simulink model "sim_tvt_2025_pos_ctrl"  (R2020a)
settings: Solver=ode4  StartTime=0.0  StopTime=30.0  FixedStep=0.01  RelTol=1e-3
values from neighbouring files (symbols this model uses):
  alfa = 0.02    [init_tvt_2025_pos_ctrl.m]
  alfa_theta = 20    [init_tvt_2025_pos_ctrl.m]
  alfa_theta_obs = 100    [init_tvt_2025_pos_ctrl.m]
  c0 = 0.1    [init_tvt_2025_pos_ctrl.m]
  c1_diff_sigma_bar_v = diag([25; 30; 20])    [init_tvt_2025_pos_ctrl.m]
  c1v = diag([5.8; 6.5; 6.5])    [init_tvt_2025_pos_ctrl.m]
  c2_diff_sigma_bar_v = diag([50; 50; 10])    [init_tvt_2025_pos_ctrl.m]
  c2v = diag([5.8; 6.5; 6.5])    [init_tvt_2025_pos_ctrl.m]
  c3_diff_sigma_bar_v = diag([15; 15; 10])    [init_tvt_2025_pos_ctrl.m]
  c3v = diag([4.8; 6.4; 6.0])    [init_tvt_2025_pos_ctrl.m]
  delta_p_i_0 = zeros(3, NF)    [init_tvt_2025_pos_ctrl.m]
  delta_v_i_0 = zeros(3, NF)    [init_tvt_2025_pos_ctrl.m]
  dp_aa_t = 0.2 * ones(3, 5) + ( 1.0 - 0.2 ) * rand(3, 5)    [init_tvt_2025_pos_ctrl.m]
  dp_ff_t = [ 0.4 * ones(1, 5) + ( 1.0 - 0.4 ) * rand(1, 5);                      0.4 * ones(1, 5) + ( 1.0 - 0.4 ) * rand(1, 5);                      0.2 * ones(1, 5) + ( 0.6 - 0.2 ) * rand(1, 5) ]    [init_tvt_2025_pos_ctrl.m]
  dp_phi_t = ( - pi / 2 ) * ones(3, 5) + ( pi / 2 - ( - pi / 2 ) ) * rand(3, 5)    [init_tvt_2025_pos_ctrl.m]
  eps0 = [0.05; 0.01; 0.01]    [init_tvt_2025_pos_ctrl.m]
  eta_ld_hat_init = zeros(3,NF)    [init_tvt_2025_pos_ctrl.m]
  etai_0 = zeros(3,5)    [init_tvt_2025_pos_ctrl.m]
  gamma0 = diag([1, 1, 1])    [init_tvt_2025_pos_ctrl.m]
  k_phi = diag([10, 10, 10])    [init_tvt_2025_pos_ctrl.m]
  k_theta = diag([5, 5, 5])    [init_tvt_2025_pos_ctrl.m]
  kai0 = [15; 10; 10]    [init_tvt_2025_pos_ctrl.m]
  kai_1_t = 0.02    [init_tvt_2025_pos_ctrl.m]
  kai_3_t = 0.1    [init_tvt_2025_pos_ctrl.m]
  ksi_ld_hat_init = zeros(3,NF)    [init_tvt_2025_pos_ctrl.m]
  ksii_0 = zeros(3,5)    [init_tvt_2025_pos_ctrl.m]
  l1v = diag([20; 20; 20])    [init_tvt_2025_pos_ctrl.m]
  l2v = diag([30; 30; 30])    [init_tvt_2025_pos_ctrl.m]
  lam0 = [15; 10; 10]    [init_tvt_2025_pos_ctrl.m]
  lam1 = diag([5,5,5])    [init_tvt_2025_pos_ctrl.m]
  lam2 = diag([5,5,5])    [init_tvt_2025_pos_ctrl.m]
  lam3 = diag([5,5,5])    [init_tvt_2025_pos_ctrl.m]
  lam4 = diag([5,5,5])    [init_tvt_2025_pos_ctrl.m]
  Lamd_diff_sigma_bar_v = 0.5    [init_tvt_2025_pos_ctrl.m]
  mass_i = zeros(1,NF)    [init_tvt_2025_pos_ctrl.m]
  Mii = diag([1;0;0;0;1])    [init_tvt_2025_pos_ctrl.m]
  pos0 = zeros(3, 1)    [init_tvt_2025_pos_ctrl.m]
  pos_bar_init = zeros(3,NF)    [init_tvt_2025_pos_ctrl.m]
  PZ0 = P0(3)    [init_tvt_2025_pos_ctrl.m]
  PZ1 = 10    [init_tvt_2025_pos_ctrl.m]
  Qci_init = repmat([1;0;0;0],1,NF)    [init_tvt_2025_pos_ctrl.m]
  R0 = 4    [init_tvt_2025_pos_ctrl.m]
  R1 = 8    [init_tvt_2025_pos_ctrl.m]
  Rx2 = 10    [init_tvt_2025_pos_ctrl.m]
  Ry2 = 6    [init_tvt_2025_pos_ctrl.m]
  Rz2 = 4    [init_tvt_2025_pos_ctrl.m]
  T0 = 0    [init_tvt_2025_pos_ctrl.m]
  T1 = tseq1    (= 10)    [init_tvt_2025_pos_ctrl.m]
  T12 = tseq1 + tseq12    (= 20)    [init_tvt_2025_pos_ctrl.m]
  T2 = tseq1 + tseq12 + tseq2    (= 30)    [init_tvt_2025_pos_ctrl.m]
  theta0 = ( 2 / 5 ) * pi    (= 1.25663706144)    [init_tvt_2025_pos_ctrl.m]
  vel0 = zeros(3, 1)    [init_tvt_2025_pos_ctrl.m]
  vel_bar_init = zeros(3,NF)    [init_tvt_2025_pos_ctrl.m]
  Wij = [0,0,1,0,0;              0,0,1,1,0;              1,0,0,0,1;              0,1,1,0,0;              0,0,1,0,0]    [init_tvt_2025_pos_ctrl.m]
  X1 = 8    [init_tvt_2025_pos_ctrl.m]
  X2 = 2    [init_tvt_2025_pos_ctrl.m]
  X3 = 3    [init_tvt_2025_pos_ctrl.m]
  Y1 = 10    [init_tvt_2025_pos_ctrl.m]
  Y2 = 2    [init_tvt_2025_pos_ctrl.m]
  Y3 = 4    [init_tvt_2025_pos_ctrl.m]
  Z1 = 4    [init_tvt_2025_pos_ctrl.m]
  Z2 = -6    [init_tvt_2025_pos_ctrl.m]
  Z3 = 2    [init_tvt_2025_pos_ctrl.m]
  zeta_diff_sigma_bar_v = 0.08    [init_tvt_2025_pos_ctrl.m]
undefined symbols (not defined in the file or in its folder): cal_frac_squ, p_alfav1, p_alfav2, p_gamma1_pos, p_gamma1_vel, p_gamma2_pos, p_gamma2_vel, q_alfav1, q_alfav2, q_gamma1_pos, q_gamma1_vel, q_gamma2_pos, q_gamma2_vel
(part 4 of 5)

== matlab function sim_tvt_2025_pos_ctrl/cal x2i agent 3 ==
  data: d_x2i_3 output; lam2 input; x2i_vec input; x3i_vec input; eta_ld_hat_vec input
function d_x2i_3 = fcn(lam2, x2i_vec, x3i_vec, eta_ld_hat_vec)
%%%% 更新高阶系统的二阶状态量
iiuav = 3;
d_x2i_3 = lam2 * ( x3i_vec(:,iiuav) - x2i_vec(:,iiuav) ) + eta_ld_hat_vec(:,iiuav);

== matlab function sim_tvt_2025_pos_ctrl/cal x2i agent 4 ==
  data: d_x2i_4 output; lam2 input; x2i_vec input; x3i_vec input; eta_ld_hat_vec input
function d_x2i_4 = fcn(lam2, x2i_vec, x3i_vec, eta_ld_hat_vec)
%%%% 更新高阶系统的二阶状态量
iiuav = 4;
d_x2i_4 = lam2 * ( x3i_vec(:,iiuav) - x2i_vec(:,iiuav) ) + eta_ld_hat_vec(:,iiuav);

== matlab function sim_tvt_2025_pos_ctrl/cal x2i agent 5 ==
  data: d_x2i_5 output; lam2 input; x2i_vec input; x3i_vec input; eta_ld_hat_vec input
function d_x2i_5 = fcn(lam2, x2i_vec, x3i_vec, eta_ld_hat_vec)
%%%% 更新高阶系统的二阶状态量
iiuav = 5;
d_x2i_5 = lam2 * ( x3i_vec(:,iiuav) - x2i_vec(:,iiuav) ) + eta_ld_hat_vec(:,iiuav);

== matlab function sim_tvt_2025_pos_ctrl/combine x2i ==
  data: x2i_1 input; x2i_vec output; x2i_2 input; x2i_3 input; x2i_4 input; x2i_5 input
function x2i_vec  = fcn(x2i_1, x2i_2, x2i_3, x2i_4, x2i_5)
%%%% 合并高阶系统的二阶状态量
x2i_vec = zeros(3,5);
x2i_vec(:,1) = x2i_1(:);
x2i_vec(:,2) = x2i_2(:);
x2i_vec(:,3) = x2i_3(:);
x2i_vec(:,4) = x2i_4(:);
x2i_vec(:,5) = x2i_5(:);

== matlab function sim_tvt_2025_pos_ctrl/cal ui agent 1 ==
  data: k_phi input; rho_hat_vec input; phi_vec input; d_phi_vec input; ui_1 output; dp_hat_vec input
function ui_1 = fcn(k_phi, rho_hat_vec, phi_vec, d_phi_vec, dp_hat_vec)
%%%% 计算控制输入ui
iiuav = 1;
g0 = 9.80663;
e3 = [0;0;1];
ui_1 = g0 * e3 + rho_hat_vec(:,iiuav) - dp_hat_vec(:,iiuav) ...
            - k_phi * ( tanh( phi_vec(:,iiuav) ) + tanh( d_phi_vec(:,iiuav) ) );

== matlab function sim_tvt_2025_pos_ctrl/cal x1i agent 1 ==
  data: d_x1i_1 output; lam1 input; x1i_vec input; x2i_vec input; eta_ld_hat_vec input
function d_x1i_1 = fcn(lam1, x1i_vec, x2i_vec, eta_ld_hat_vec)
%%%% 更新高阶系统的一阶状态量
iiuav = 1;
d_x1i_1 = lam1 * ( x2i_vec(:,iiuav) - x1i_vec(:,iiuav) ) + eta_ld_hat_vec(:,iiuav);

== matlab function sim_tvt_2025_pos_ctrl/cal x1i agent 2 ==
  data: d_x1i_2 output; lam1 input; x1i_vec input; x2i_vec input; eta_ld_hat_vec input
function d_x1i_2 = fcn(lam1, x1i_vec, x2i_vec, eta_ld_hat_vec)
%%%% 更新高阶系统的一阶状态量
iiuav = 2;
d_x1i_2 = lam1 * ( x2i_vec(:,iiuav) - x1i_vec(:,iiuav) ) + eta_ld_hat_vec(:,iiuav);

== matlab function sim_tvt_2025_pos_ctrl/cal x1i agent 3 ==
  data: d_x1i_3 output; lam1 input; x1i_vec input; x2i_vec input; eta_ld_hat_vec input
function d_x1i_3 = fcn(lam1, x1i_vec, x2i_vec, eta_ld_hat_vec)
%%%% 更新高阶系统的一阶状态量
iiuav = 3;
d_x1i_3 = lam1 * ( x2i_vec(:,iiuav) - x1i_vec(:,iiuav) ) + eta_ld_hat_vec(:,iiuav);

== matlab function sim_tvt_2025_pos_ctrl/cal x1i agent 4 ==
  data: d_x1i_4 output; lam1 input; x1i_vec input; x2i_vec input; eta_ld_hat_vec input
function d_x1i_4 = fcn(lam1, x1i_vec, x2i_vec, eta_ld_hat_vec)
%%%% 更新高阶系统的一阶状态量
iiuav = 4;
d_x1i_4 = lam1 * ( x2i_vec(:,iiuav) - x1i_vec(:,iiuav) ) + eta_ld_hat_vec(:,iiuav);

== matlab function sim_tvt_2025_pos_ctrl/combine ui ==
  data: ui_1 input; ui_2 input; ui_3 input; ui_4 input; ui_5 input; ui output
function ui  = fcn(ui_1, ui_2, ui_3, ui_4, ui_5)
%%%% 合并控制输入ui
ui = [ui_1(:), ui_2(:), ui_3(:), ui_4(:), ui_5(:)];

== matlab function sim_tvt_2025_pos_ctrl/update sigmai agent 1 ==
  data: kai0 input; lam0 input; eps0 input; d_sigmai_1 output; Wij input; Mii input; tsim input; u0 input; beta_hat_vec input; rho_hat_vec input; Phi_sec_sigma_vec input
function d_sigmai_1 = fcn(kai0, lam0, eps0, Wij, Mii, tsim, u0, beta_hat_vec, rho_hat_vec, Phi_sec_sigma_vec)
%%%% 求解分布式观测器变量
iiuav = 1;
err_rho = Mii(iiuav, iiuav) * ( rho_hat_vec(:,iiuav) - u0(:) );
for jjuav = 1:5
    err_rho = err_rho + Wij(iiuav, jjuav) * ( rho_hat_vec(:,iiuav) - rho_hat_vec(:,jjuav) );
end
d_sigmai_1 = -inv( Phi_sec_sigma_vec(:,:,iiuav) ) * ( ( kai0(:) ./ lam0(:) ) .* err_rho(:) ...
                                + ( beta_hat_vec(iiuav) ./ lam0(:) ) .* tanh( err_rho(:) ./ exp( -eps0 * tsim ) ) );

== matlab function sim_tvt_2025_pos_ctrl/cal disturbance observation error dp_tilt ==
  data: dp_vec input; dp_tilt_vec output; dp_hat_vec input
function dp_tilt_vec = fcn(dp_vec, dp_hat_vec)
%%%% 计算扰动观测器估计误差dp_tilt
dp_tilt_vec = zeros(3,5);
for iiuav = 1:5
    dp_tilt_vec(:,iiuav) = dp_vec(:,iiuav) - dp_hat_vec(:,iiuav);
end

== matlab function sim_tvt_2025_pos_ctrl/leader control input ==
  data: t input; u0 output; T1 input; T2 input; R0 input; R1 input; Rx2 input; Ry2 input; Rz2 input
function u0  = fcn(t, T1, T2, R0, R1, Rx2, Ry2, Rz2)
%%%% 给出领导者参考加速度控制输入
u0 = zeros(3, 1);

if t <= ( T1 + 1e-05 )
    u0(1, 1) = - ( 4 * pi * sin( ( 2 * pi * ( t - 0 ) ) / ( 0 - T1 ) ) * ( R0 - R1 ) ) / ( ( 0 - T1 ) ^ 2 ) ...
                        - ( 4 * ( pi ^ 2 ) * cos( ( 2 * pi * ( t - 0 ) ) / ( 0 - T1 ) ) ...
                        * ( R0 + ( ( R0 - R1 ) * ( t - 0 ) ) / ( 0 - T1 ) ) ) / ( ( 0 - T1 ) ^ 2 );
    u0(2, 1) = ( 4 * pi * cos( ( 2 * pi * ( t - 0 ) ) / ( 0 - T1 ) ) * ( R0 - R1 ) ) / ( ( 0 - T1 ) ^ 2 ) ...
                        - ( 4 * ( pi ^ 2 ) * sin( ( 2 * pi * ( t - 0 ) ) / ( 0 - T1 ) ) ...
                        * ( R0 + ( ( R0 - R1 ) * ( t - 0 ) ) / ( 0 - T1 ) ) ) / ( ( 0 - T1 ) ^ 2 );
    u0(3, 1) = 0;
else
    u0(1, 1) = ( 4 * Rx2 * ( pi ^ 2 ) * cos( ( 2 * pi * ( t - T1 ) ) / ( T1 - T2 ) ) ) / ( ( T1 - T2 ) ^ 2 );
    u0(2, 1) = - ( 16 * Ry2 * ( pi ^ 2 ) * sin( ( 4 * pi * ( t - T1 ) ) / ( T1 - T2 ) ) ) / ( ( T1 - T2 ) ^ 2 );
    u0(3, 1) = ( 16 * Rz2 * ( pi ^ 2 ) * sin( ( 4 * pi * ( t - T1 ) ) / ( T1 - T2 ) ) ) / ( ( T1 - T2 ) ^ 2 );
end

== matlab function sim_tvt_2025_pos_ctrl/process velocity ==
  data: T0 input; T1 input; T2 input; PZ0 input; PZ1 input; R0 input; R1 input; Rx2 input; Ry2 input; Rz2 input; t input; V_init_out output
function V_init_out = fcn(T0, T1, T2, PZ0, PZ1, R0, R1, Rx2, Ry2, Rz2, t)
V_init_out = zeros(3, 1);
if t < T1 + 1e-05
    V_init_out(1, 1) = ( cos( ( 2 * pi * ( t - T0 ) ) / ( T0 - T1 ) ) * ( R0 - R1 ) ) / ( T0 - T1 ) ...
                                    - ( 2 * pi * sin( ( 2 * pi * ( t - T0 ) ) / ( T0 - T1 ) ) * ( R0 + ( ( R0 - R1 ) * ( t - T0 ) ) / ( T0 - T1 ) ) ) / ( T0 - T1 );
    V_init_out(2, 1) = ( sin( ( 2 * pi * ( t - T0 ) ) / ( T0 - T1 ) ) * ( R0 - R1 ) ) / ( T0 - T1 ) ...
                                    + ( 2 * pi * cos( ( 2 * pi * ( t - T0 ) ) / ( T0 - T1 ) ) * ( R0 + ( ( R0 - R1 ) * ( t - T0 ) ) / ( T0 - T1 ) ) ) / ( T0 - T1 );
    V_init_out(3, 1) = ( PZ0 - PZ1 ) / ( T0 - T1 );
else
    V_init_out(1, 1) = ( 2 * Rx2 * pi * sin( ( 2 * pi * ( t - T1 ) ) / ( T1 - T2 ) ) ) / ( T1 - T2 );
    V_init_out(2, 1) = ( 4 * Ry2 * pi * cos( ( 4 * pi * ( t - T1 ) ) / ( T1 - T2 ) ) ) / ( T1 - T2 );
    V_init_out(3, 1) = - ( 4 * Rz2 * pi * cos( ( 4 * pi * ( t - T1 ) ) / ( T1 - T2 ) ) ) / ( T1 - T2 );
end

== matlab function sim_tvt_2025_pos_ctrl/set desire formation configuration ==
  data: X1 input; X2 input; X3 input; Y1 input; Y2 input; Y3 input; Z1 input; Z2 input; Z3 input; theta0 input; kai_1_t input; kai_3_t input; T1 input; T12 input; t input; delta_ksi_vec output; delta_eta_vec output; d_delta_eta_vec output
function [delta_ksi_vec, delta_eta_vec, d_delta_eta_vec] = fcn(X1, X2, X3, Y1, Y2, Y3, Z1, Z2, Z3, ...
                                                                                                                theta0, kai_1_t, kai_3_t, T1, T12, t)
%%%% 计算跟随者期望速度分布式观测器误差
delta_ksi_vec = zeros(3, 5);
delta_eta_vec = zeros(3, 5);
d_delta_eta_vec = zeros(3, 5);
if t <= ( T1 + 1e-04 )
    exp_tmp = exp( -kai_1_t * t );
    delta_ksi_vec(:, 1) = [ X1 * cos( theta0 ) - X2 * exp_tmp; ...
                                            Y1 * sin( theta0 ) - Y2 * exp_tmp; ...
                                            Z1 - Z2 * exp_tmp ];
    delta_ksi_vec(:, 2) = [ - X1 * cos( theta0 ) + X2 * exp_tmp; ...
                                            Y1 * sin( theta0 ) - Y2 * exp_tmp; ...
                                            Z1 + Z2 * exp_tmp ];
    delta_ksi_vec(:, 3) = [ X1 - X2 * exp_tmp; ...
                                            Y2 * exp_tmp; ...
                                            ( 3 / 8 ) * Z1 + Z2 * exp_tmp ];
    delta_ksi_vec(:, 4) = [ - X1 * cos( theta0 ) + X2 * exp_tmp; ...
                                            - Y1 * sin( theta0 ) + Y2 * exp_tmp; ...
                                            Z1 + Z2 * exp_tmp ];
    delta_ksi_vec(:, 5) = [ X1 * cos( theta0 ) - X2 * exp_tmp; ...
                                            - Y1 * sin( theta0 ) + Y2 * exp_tmp; ...
                                            Z1 - Z2 * exp_tmp ];
    delta_eta_vec(:, 1) = [ kai_1_t * X2 * exp_tmp; kai_1_t * Y2 * exp_tmp; kai_1_t * Z2 * exp_tmp ];
    delta_eta_vec(:, 2) = [ - kai_1_t * X2 * exp_tmp; kai_1_t * Y2 * exp_tmp; - kai_1_t * Z2 * exp_tmp ];
    delta_eta_vec(:, 3) = [ kai_1_t * X2 * exp_tmp; - kai_1_t * Y2 * exp_tmp; - kai_1_t * Z2 * exp_tmp ];
    delta_eta_vec(:, 4) = [ - kai_1_t * X2 * exp_tmp; - kai_1_t * Y2 * exp_tmp; - kai_1_t * Z2 * exp_tmp ];
    delta_eta_vec(:, 5) = [ kai_1_t * X2 * exp_tmp; - kai_1_t * Y2 * exp_tmp; kai_1_t * Z2 * exp_tmp ];
    d_delta_eta_vec(:, 1) = [ - ( kai_1_t ^ 2 ) * X2 * exp_tmp; - ( kai_1_t ^ 2 ) * Y2 * exp_tmp; - ( kai_1_t ^ 2 ) * Z2 * exp_tmp ];
    d_delta_eta_vec(:, 2) = [ ( kai_1_t ^ 2 ) * X2 * exp_tmp; - ( kai_1_t ^ 2 ) * Y2 * exp_tmp; ( kai_1_t ^ 2 ) * Z2 * exp_tmp ];
    d_delta_eta_vec(:, 3) = [ - ( kai_1_t ^ 2 ) * X2 * exp_tmp; ( kai_1_t ^ 2 ) * Y2 * exp_tmp; ( kai_1_t ^ 2 ) * Z2 * exp_tmp ];
    d_delta_eta_vec(:, 4) = [ ( kai_1_t ^ 2 ) * X2 * exp_tmp; ( kai_1_t ^ 2 ) * Y2 * exp_tmp; ( kai_1_t ^ 2 ) * Z2 * exp_tmp ];
    d_delta_eta_vec(:, 5) = [ - ( kai_1_t ^ 2 ) * X2 * exp_tmp; ( kai_1_t ^ 2 ) * Y2 * exp_tmp; - ( kai_1_t ^ 2 ) * Z2 * exp_tmp ];
elseif t <= ( T12 + 1e-04 )
    delta_ksi_vec(:, 1) = [ X1 * cos( theta0 ) - X2; Y1 * sin( theta0 ) - Y2; Z1 - Z2 ];
    delta_ksi_vec(:, 2) = [ - X1 * cos( theta0 ) + X2; Y1 * sin( theta0 ) - Y2; Z1 + Z2 ];
    delta_ksi_vec(:, 3) = [ X1 - X2; 0; ( 3 / 8 ) * Z1 + Z2 ];
    delta_ksi_vec(:, 4) = [ - X1 * cos( theta0 ) + X2; - Y1 * sin( theta0 ) + Y2; Z1 + Z2 ];
    delta_ksi_vec(:, 5) = [ X1 * cos( theta0 ) - X2; - Y1 * sin( theta0 ) + Y2; Z1 - Z2 ];
else
    exp_tmp = 1 / ( 1 + exp( - kai_3_t * ( t - T12 - 5 ) ) );
    tmp_2 = exp( - kai_3_t * ( t - T12 - 5 ) ) / ( ( 1 + exp( - kai_3_t * ( t - T12 - 5 ) ) ) ^ 2 );
    delta_ksi_vec(:, 1) = [ X1 * cos( theta0 ) - X2 + X3 * exp_tmp; ...
                                            Y1 * sin( theta0 ) - Y2 + Y3 * exp_tmp; ...
                                            Z1 - Z2 + Z3 * exp_tmp ];
    delta_ksi_vec(:, 2) = [ - X1 * cos( theta0 ) + X2 - X3 * exp_tmp; ...
                                            Y1 * sin( theta0 ) - Y2 + Y3 * exp_tmp; ...
                                            Z1 + Z2 - Z3 * exp_tmp ];
    delta_ksi_vec(:, 3) = [ X1 - X2 + X3 * exp_tmp; ...
                                            - Y3 * exp_tmp; ...
                                            ( 3 / 8 ) * Z1 + Z2 - Z3 * exp_tmp ];
    delta_ksi_vec(:, 4) = [ - X1 * cos( theta0 ) + X2 - X3 * exp_tmp; ...
                                            - Y1 * sin( theta0 ) + Y2 - Y3 * exp_tmp; ...
                                            Z1 + Z2 - Z3 * exp_tmp ];
    delta_ksi_vec(:, 5) = [ X1 * cos( theta0 ) - X2 + X3 * exp_tmp; ...
                                            - Y1 * sin( theta0 ) + Y2 - Y3 * exp_tmp; ...
                                            Z1 - Z2 + Z3 * exp_tmp ];
    delta_eta_vec(:, 1) = [ kai_3_t * X3 * tmp_2; kai_3_t * Y3 * tmp_2; kai_3_t * Z3 * tmp_2 ];
    delta_eta_vec(:, 2) = [ - kai_3_t * X3 * tmp_2; kai_3_t * Y3 * tmp_2; kai_3_t * Z3 * tmp_2 ];
    delta_eta_vec(:, 3) = [ kai_3_t * X3 * tmp_2; - kai_3_t * Y3 * tmp_2; - kai_3_t * Z3 * tmp_2 ];
    delta_eta_vec(:, 4) = [ - kai_3_t * X3 * tmp_2; - kai_3_t * Y3 * tmp_2; - kai_3_t * Z3 * tmp_2 ];
    delta_eta_vec(:, 5) = [ kai_3_t * X3 * tmp_2; kai_3_t * Y3 * tmp_2; - kai_3_t * Z3 * tmp_2 ];
    d_delta_eta_vec(:, 1) = ( kai_3_t * ( 1 - exp( - kai_3_t * ( t - T12 - 5 ) ) ) * exp_tmp ) * delta_eta_vec(:, 1);
    d_delta_eta_vec(:, 2) = ( kai_3_t * ( 1 - exp( - kai_3_t * ( t - T12 - 5 ) ) ) * exp_tmp ) * delta_eta_vec(:, 2);
    d_delta_eta_vec(:, 3) = ( kai_3_t * ( 1 - exp( - kai_3_t * ( t - T12 - 5 ) ) ) * exp_tmp ) * delta_eta_vec(:, 3);
    d_delta_eta_vec(:, 4) = ( kai_3_t * ( 1 - exp( - kai_3_t * ( t - T12 - 5 ) ) ) * exp_tmp ) * delta_eta_vec(:, 4);
    d_delta_eta_vec(:, 5) = ( kai_3_t * ( 1 - exp( - kai_3_t * ( t - T12 - 5 ) ) ) * exp_tmp ) * delta_eta_vec(:, 5);
end

== matlab function sim_tvt_2025_pos_ctrl/cal x1i agent 5 ==
  data: d_x1i_5 output; lam1 input; x1i_vec input; x2i_vec input; eta_ld_hat_vec input
function d_x1i_5 = fcn(lam1, x1i_vec, x2i_vec, eta_ld_hat_vec)
%%%% 更新高阶系统的一阶状态量
iiuav = 5;
d_x1i_5 = lam1 * ( x2i_vec(:,iiuav) - x1i_vec(:,iiuav) ) + eta_ld_hat_vec(:,iiuav);

== matlab function sim_tvt_2025_pos_ctrl/combine x1i ==
  data: x1i_1 input; x1i_vec output; x1i_2 input; x1i_3 input; x1i_4 input; x1i_5 input
function x1i_vec  = fcn(x1i_1, x1i_2, x1i_3, x1i_4, x1i_5)
%%%% 合并高阶系统的一阶状态量
x1i_vec = zeros(3,5);
x1i_vec(:,1) = x1i_1(:);
x1i_vec(:,2) = x1i_2(:);
x1i_vec(:,3) = x1i_3(:);
x1i_vec(:,4) = x1i_4(:);
x1i_vec(:,5) = x1i_5(:);

== matlab function sim_tvt_2025_pos_ctrl/cal yi ==
  data: x1i_vec input; yi_vec output
function yi_vec  = fcn(x1i_vec)
%%%% 得到高阶系统输出
yi_vec = zeros(3,5);
for iiuav = 1:5
    yi_vec(:,iiuav) = x1i_vec(:,iiuav);
end

== matlab function sim_tvt_2025_pos_ctrl/cal betai agent 1 ==
  data: betai_1 output; gamma0 input; pos_bar_vec input; yi_vec input
function betai_1 = fcn(gamma0, pos_bar_vec, yi_vec)
%%%% 更新辅助变量
iiuav = 1;
betai_1 = -gamma0 * ( pos_bar_vec(:,iiuav) - yi_vec(:,iiuav) );

== matlab function sim_tvt_2025_pos_ctrl/cal betai agent 2 ==
  data: betai_2 output; gamma0 input; pos_bar_vec input; yi_vec input
function betai_2 = fcn(gamma0, pos_bar_vec, yi_vec)
%%%% 更新辅助变量
iiuav = 2;
betai_2 = -gamma0 * ( pos_bar_vec(:,iiuav) - yi_vec(:,iiuav) );

== matlab function sim_tvt_2025_pos_ctrl/cal betai agent 3 ==
  data: betai_3 output; gamma0 input; pos_bar_vec input; yi_vec input
function betai_3 = fcn(gamma0, pos_bar_vec, yi_vec)
%%%% 更新辅助变量
iiuav = 3;
betai_3 = -gamma0 * ( pos_bar_vec(:,iiuav) - yi_vec(:,iiuav) );

== matlab function sim_tvt_2025_pos_ctrl/cal betai agent 4 ==
  data: betai_4 output; gamma0 input; pos_bar_vec input; yi_vec input
function betai_4 = fcn(gamma0, pos_bar_vec, yi_vec)
%%%% 更新辅助变量
iiuav = 4;
betai_4 = -gamma0 * ( pos_bar_vec(:,iiuav) - yi_vec(:,iiuav) );

== matlab function sim_tvt_2025_pos_ctrl/cal betai agent 5 ==
  data: betai_5 output; gamma0 input; pos_bar_vec input; yi_vec input
function betai_5 = fcn(gamma0, pos_bar_vec, yi_vec)
%%%% 更新辅助变量
iiuav = 5;
betai_5 = -gamma0 * ( pos_bar_vec(:,iiuav) - yi_vec(:,iiuav) );

== matlab function sim_tvt_2025_pos_ctrl/combine beta ==
  data: beta_1 input; beta_vec output; beta_2 input; beta_3 input; beta_4 input; beta_5 input
function beta_vec  = fcn(beta_1, beta_2, beta_3, beta_4, beta_5)
%%%% 合并辅助变量
beta_vec = zeros(3,5);
beta_vec(:,1) = beta_1(:);
beta_vec(:,2) = beta_2(:);
beta_vec(:,3) = beta_3(:);
beta_vec(:,4) = beta_4(:);
beta_vec(:,5) = beta_5(:);

== matlab function sim_tvt_2025_pos_ctrl/cal thetai agent 1 ==
  data: thetai_1 output; k_theta input; err_vel_vec input; beta_vec input; d_beta_vec input
function thetai_1 = fcn(k_theta, err_vel_vec, beta_vec, d_beta_vec)
%%%% 更新辅助变量
iiuav = 1;
thetai_1 = k_theta * ( ( err_vel_vec(:,iiuav) - beta_vec(:,iiuav) ) - d_beta_vec(:,iiuav) );

== matlab function sim_tvt_2025_pos_ctrl/update sigmai agent 2 ==
  data: kai0 input; lam0 input; eps0 input; d_sigmai_2 output; Wij input; Mii input; tsim input; u0 input; beta_hat_vec input; rho_hat_vec input; Phi_sec_sigma_vec input
function d_sigmai_2 = fcn(kai0, lam0, eps0, Wij, Mii, tsim, u0, beta_hat_vec, rho_hat_vec, Phi_sec_sigma_vec)
%%%% 求解分布式观测器变量
iiuav = 2;
err_rho = Mii(iiuav, iiuav) * ( rho_hat_vec(:,iiuav) - u0(:) );
for jjuav = 1:5
    err_rho = err_rho + Wij(iiuav, jjuav) * ( rho_hat_vec(:,iiuav) - rho_hat_vec(:,jjuav) );
end
d_sigmai_2 = -inv( Phi_sec_sigma_vec(:,:,iiuav) ) * ( ( kai0(:) ./ lam0(:) ) .* err_rho(:) ...
                                + ( beta_hat_vec(iiuav) ./ lam0(:) ) .* tanh( err_rho(:) ./ exp( -eps0 * tsim ) ) );

== matlab function sim_tvt_2025_pos_ctrl/combine d_xi1 ==
  data: d_x1i_1 input; d_x1i_vec output; d_x1i_2 input; d_x1i_3 input; d_x1i_4 input; d_x1i_5 input
function d_x1i_vec  = fcn(d_x1i_1, d_x1i_2, d_x1i_3, d_x1i_4, d_x1i_5)
%%%% 合并高阶系统的一阶状态量导数
d_x1i_vec = zeros(3,5);
d_x1i_vec(:,1) = d_x1i_1(:);
d_x1i_vec(:,2) = d_x1i_2(:);
d_x1i_vec(:,3) = d_x1i_3(:);
d_x1i_vec(:,4) = d_x1i_4(:);
d_x1i_vec(:,5) = d_x1i_5(:);

== matlab function sim_tvt_2025_pos_ctrl/cal d_yi ==
  data: d_x1i_vec input; d_yi_vec output
function d_yi_vec  = fcn(d_x1i_vec)
%%%% 得到高阶系统输出的导数
d_yi_vec = zeros(3,5);
for iiuav = 1:5
    d_yi_vec(:,iiuav) = d_x1i_vec(:,iiuav);
end

== matlab function sim_tvt_2025_pos_ctrl/cal d_betai agent 1 ==
  data: d_betai_1 output; gamma0 input; eta_i_vec input; d_phi_vec input; d_yi_vec input
function d_betai_1 = fcn(gamma0, eta_i_vec, d_phi_vec, d_yi_vec)
%%%% 更新辅助变量导数
iiuav = 1;
d_betai_1 = -gamma0 * ( eta_i_vec(:,iiuav) - d_phi_vec(:,iiuav) - d_yi_vec(:,iiuav) );

== matlab function sim_tvt_2025_pos_ctrl/cal d_betai agent 2 ==
  data: d_betai_2 output; gamma0 input; eta_i_vec input; d_phi_vec input; d_yi_vec input
function d_betai_2 = fcn(gamma0, eta_i_vec, d_phi_vec, d_yi_vec)
%%%% 更新辅助变量导数
iiuav = 2;
d_betai_2 = -gamma0 * ( eta_i_vec(:,iiuav) - d_phi_vec(:,iiuav) - d_yi_vec(:,iiuav) );

== matlab function sim_tvt_2025_pos_ctrl/cal d_betai agent 3 ==
  data: d_betai_3 output; gamma0 input; eta_i_vec input; d_phi_vec input; d_yi_vec input
function d_betai_3 = fcn(gamma0, eta_i_vec, d_phi_vec, d_yi_vec)
%%%% 更新辅助变量导数
iiuav = 3;
d_betai_3 = -gamma0 * ( eta_i_vec(:,iiuav) - d_phi_vec(:,iiuav) - d_yi_vec(:,iiuav) );

== matlab function sim_tvt_2025_pos_ctrl/cal d_betai agent 4 ==
  data: d_betai_4 output; gamma0 input; eta_i_vec input; d_phi_vec input; d_yi_vec input
function d_betai_4 = fcn(gamma0, eta_i_vec, d_phi_vec, d_yi_vec)
%%%% 更新辅助变量导数
iiuav = 4;
d_betai_4 = -gamma0 * ( eta_i_vec(:,iiuav) - d_phi_vec(:,iiuav) - d_yi_vec(:,iiuav) );

== matlab function sim_tvt_2025_pos_ctrl/cal d_betai agent 5 ==
  data: d_betai_5 output; gamma0 input; eta_i_vec input; d_phi_vec input; d_yi_vec input
function d_betai_5 = fcn(gamma0, eta_i_vec, d_phi_vec, d_yi_vec)
%%%% 更新辅助变量导数
iiuav = 5;
d_betai_5 = -gamma0 * ( eta_i_vec(:,iiuav) - d_phi_vec(:,iiuav) - d_yi_vec(:,iiuav) );

== matlab function sim_tvt_2025_pos_ctrl/combine d_betai ==
  data: d_beta_1 input; d_beta_vec output; d_beta_2 input; d_beta_3 input; d_beta_4 input; d_beta_5 input
function d_beta_vec  = fcn(d_beta_1, d_beta_2, d_beta_3, d_beta_4, d_beta_5)
%%%% 合并辅助变量导数
d_beta_vec = zeros(3,5);
d_beta_vec(:,1) = d_beta_1(:);
d_beta_vec(:,2) = d_beta_2(:);
d_beta_vec(:,3) = d_beta_3(:);
d_beta_vec(:,4) = d_beta_4(:);
d_beta_vec(:,5) = d_beta_5(:);

== matlab function sim_tvt_2025_pos_ctrl/cal thetai agent 2 ==
  data: thetai_2 output; k_theta input; err_vel_vec input; beta_vec input; d_beta_vec input
function thetai_2 = fcn(k_theta, err_vel_vec, beta_vec, d_beta_vec)
%%%% 更新辅助变量
iiuav = 2;
thetai_2 = k_theta * ( ( err_vel_vec(:,iiuav) - beta_vec(:,iiuav) ) - d_beta_vec(:,iiuav) );

== matlab function sim_tvt_2025_pos_ctrl/cal thetai agent 3 ==
  data: thetai_3 output; k_theta input; err_vel_vec input; beta_vec input; d_beta_vec input
function thetai_3 = fcn(k_theta, err_vel_vec, beta_vec, d_beta_vec)
%%%% 更新辅助变量
iiuav = 3;
thetai_3 = k_theta * ( ( err_vel_vec(:,iiuav) - beta_vec(:,iiuav) ) - d_beta_vec(:,iiuav) );

== matlab function sim_tvt_2025_pos_ctrl/cal thetai agent 4 ==
  data: thetai_4 output; k_theta input; err_vel_vec input; beta_vec input; d_beta_vec input
function thetai_4 = fcn(k_theta, err_vel_vec, beta_vec, d_beta_vec)
%%%% 更新辅助变量
iiuav = 4;
thetai_4 = k_theta * ( ( err_vel_vec(:,iiuav) - beta_vec(:,iiuav) ) - d_beta_vec(:,iiuav) );

== matlab function sim_tvt_2025_pos_ctrl/cal thetai agent 5 ==
  data: thetai_5 output; k_theta input; err_vel_vec input; beta_vec input; d_beta_vec input
function thetai_5 = fcn(k_theta, err_vel_vec, beta_vec, d_beta_vec)
%%%% 更新辅助变量
iiuav = 5;
thetai_5 = k_theta * ( ( err_vel_vec(:,iiuav) - beta_vec(:,iiuav) ) - d_beta_vec(:,iiuav) );

== matlab function sim_tvt_2025_pos_ctrl/combine thetai ==
  data: theta_1 input; theta_vec output; theta_2 input; theta_3 input; theta_4 input; theta_5 input
function theta_vec  = fcn(theta_1, theta_2, theta_3, theta_4, theta_5)
%%%% 合并辅助变量
theta_vec = zeros(3,5);
theta_vec(:,1) = theta_1(:);
theta_vec(:,2) = theta_2(:);
theta_vec(:,3) = theta_3(:);
theta_vec(:,4) = theta_4(:);
theta_vec(:,5) = theta_5(:);

== matlab function sim_tvt_2025_pos_ctrl/cal phi agent 1 ==
  data: d2_phi_1 output; k_phi input; phi_vec input; d_phi_vec input; theta_vec input
function d2_phi_1 = fcn(k_phi, phi_vec, d_phi_vec, theta_vec)
%%%% 更新辅助变量的二阶导数
iiuav = 1;
d2_phi_1 = -k_phi * ( tanh( phi_vec(:,iiuav) ) + tanh( d_phi_vec(:,iiuav) ) ) + theta_vec(:,iiuav);

== matlab function sim_tvt_2025_pos_ctrl/cal phi agent 2 ==
  data: d2_phi_2 output; k_phi input; phi_vec input; d_phi_vec input; theta_vec input
function d2_phi_2 = fcn(k_phi, phi_vec, d_phi_vec, theta_vec)
%%%% 更新辅助变量的二阶导数
iiuav = 2;
d2_phi_2 = -k_phi * ( tanh( phi_vec(:,iiuav) ) + tanh( d_phi_vec(:,iiuav) ) ) + theta_vec(:,iiuav);

== matlab function sim_tvt_2025_pos_ctrl/cal phi agent 3 ==
  data: d2_phi_3 output; k_phi input; phi_vec input; d_phi_vec input; theta_vec input
function d2_phi_3 = fcn(k_phi, phi_vec, d_phi_vec, theta_vec)
%%%% 更新辅助变量的二阶导数
iiuav = 3;
d2_phi_3 = -k_phi * ( tanh( phi_vec(:,iiuav) ) + tanh( d_phi_vec(:,iiuav) ) ) + theta_vec(:,iiuav);

== matlab function sim_tvt_2025_pos_ctrl/update sigmai agent 3 ==
  data: kai0 input; lam0 input; eps0 input; d_sigmai_3 output; Wij input; Mii input; tsim input; u0 input; beta_hat_vec input; rho_hat_vec input; Phi_sec_sigma_vec input
function d_sigmai_3 = fcn(kai0, lam0, eps0, Wij, Mii, tsim, u0, beta_hat_vec, rho_hat_vec, Phi_sec_sigma_vec)
%%%% 求解分布式观测器变量
iiuav = 3;
err_rho = Mii(iiuav, iiuav) * ( rho_hat_vec(:,iiuav) - u0(:) );
for jjuav = 1:5
    err_rho = err_rho + Wij(iiuav, jjuav) * ( rho_hat_vec(:,iiuav) - rho_hat_vec(:,jjuav) );
end
d_sigmai_3 = -inv( Phi_sec_sigma_vec(:,:,iiuav) ) * ( ( kai0(:) ./ lam0(:) ) .* err_rho(:) ...
                                + ( beta_hat_vec(iiuav) ./ lam0(:) ) .* tanh( err_rho(:) ./ exp( -eps0 * tsim ) ) );

== matlab function sim_tvt_2025_pos_ctrl/cal phi agent 4 ==
  data: d2_phi_4 output; k_phi input; phi_vec input; d_phi_vec input; theta_vec input
function d2_phi_4 = fcn(k_phi, phi_vec, d_phi_vec, theta_vec)
%%%% 更新辅助变量的二阶导数
iiuav = 4;
d2_phi_4 = -k_phi * ( tanh( phi_vec(:,iiuav) ) + tanh( d_phi_vec(:,iiuav) ) ) + theta_vec(:,iiuav);

== matlab function sim_tvt_2025_pos_ctrl/cal phi agent 5 ==
  data: d2_phi_5 output; k_phi input; phi_vec input; d_phi_vec input; theta_vec input
function d2_phi_5 = fcn(k_phi, phi_vec, d_phi_vec, theta_vec)
%%%% 更新辅助变量的二阶导数
iiuav = 5;
d2_phi_5 = -k_phi * ( tanh( phi_vec(:,iiuav) ) + tanh( d_phi_vec(:,iiuav) ) ) + theta_vec(:,iiuav);

== matlab function sim_tvt_2025_pos_ctrl/combine d_phi ==
  data: d_phi_1 input; d_phi_vec output; d_phi_2 input; d_phi_3 input; d_phi_4 input; d_phi_5 input
function d_phi_vec  = fcn(d_phi_1, d_phi_2, d_phi_3, d_phi_4, d_phi_5)
%%%% 合并辅助变量一阶导数
d_phi_vec = zeros(3,5);
d_phi_vec(:,1) = d_phi_1(:);
d_phi_vec(:,2) = d_phi_2(:);
d_phi_vec(:,3) = d_phi_3(:);
d_phi_vec(:,4) = d_phi_4(:);
d_phi_vec(:,5) = d_phi_5(:);

== matlab function sim_tvt_2025_pos_ctrl/combine phi ==
  data: phi_1 input; phi_vec output; phi_2 input; phi_3 input; phi_4 input; phi_5 input
function phi_vec  = fcn(phi_1, phi_2, phi_3, phi_4, phi_5)
%%%% 合并辅助变量
phi_vec = zeros(3,5);
phi_vec(:,1) = phi_1(:);
phi_vec(:,2) = phi_2(:);
phi_vec(:,3) = phi_3(:);
phi_vec(:,4) = phi_4(:);
phi_vec(:,5) = phi_5(:);

== matlab function sim_tvt_2025_pos_ctrl/cal abs 56 ==
  data: x input; y output
function y = fcn(x)
y = abs(x(:));

== matlab function sim_tvt_2025_pos_ctrl/cal abs 57 ==
  data: x input; y output
function y = fcn(x)
y = abs(x(:));

== matlab function sim_tvt_2025_pos_ctrl/cal abs 58 ==
  data: x input; y output
function y = fcn(x)
y = abs(x(:));

== matlab function sim_tvt_2025_pos_ctrl/cal abs 59 ==
  data: x input; y output
function y = fcn(x)
y = abs(x(:));

== matlab function sim_tvt_2025_pos_ctrl/cal abs 60 ==
  data: x input; y output
function y = fcn(x)
y = abs(x(:));

== matlab function sim_tvt_2025_pos_ctrl/cal lumped observation error agent 1 ==
  data: wij input; w0 input; ksi_d_est_vec input; ksi0 input; delta_ksi_vec input; eta_d_est_vec input; ksi_est_err_tilt_1 output; eta0 input; delta_eta_vec input; eta_est_err_tilt_1 output
function [ksi_est_err_tilt_1, eta_est_err_tilt_1]  = fcn(wij, w0, ksi_d_est_vec, ksi0, delta_ksi_vec, eta_d_est_vec, eta0, delta_eta_vec)
%%%% 计算跟随者期望速度分布式观测器误差
iiuav = 1;
ksi_est_err_tilt_1 = w0(iiuav, iiuav) * (ksi_d_est_vec(:,iiuav) - ksi0(:) - delta_ksi_vec(:,iiuav));
eta_est_err_tilt_1 = w0(iiuav, iiuav) * (eta_d_est_vec(:,iiuav) - eta0(:) - delta_eta_vec(:,iiuav));
for jjuav = 1:5
    ksi_est_err_tilt_1 = ksi_est_err_tilt_1 + ...
                                        wij(iiuav, jjuav) * ((ksi_d_est_vec(:,iiuav) - delta_ksi_vec(:,iiuav)) - (ksi_d_est_vec(:,jjuav) - delta_ksi_vec(:,jjuav)));
    eta_est_err_tilt_1 = eta_est_err_tilt_1 + ...
                                        wij(iiuav, jjuav) * ((eta_d_est_vec(:,iiuav) - delta_eta_vec(:,iiuav)) - (eta_d_est_vec(:,jjuav) - delta_eta_vec(:,jjuav)));
end

== matlab function sim_tvt_2025_pos_ctrl/cal lumped observation error agent 2 ==
  data: wij input; w0 input; ksi_d_est_vec input; ksi0 input; delta_ksi_vec input; eta_d_est_vec input; ksi_est_err_tilt_2 output; eta0 input; delta_eta_vec input; eta_est_err_tilt_2 output
function [ksi_est_err_tilt_2, eta_est_err_tilt_2]  = fcn(wij, w0, ksi_d_est_vec, ksi0, delta_ksi_vec, eta_d_est_vec, eta0, delta_eta_vec)
%%%% 计算跟随者期望速度分布式观测器误差
iiuav = 2;
ksi_est_err_tilt_2 = w0(iiuav, iiuav) * (ksi_d_est_vec(:,iiuav) - ksi0(:) - delta_ksi_vec(:,iiuav));
eta_est_err_tilt_2 = w0(iiuav, iiuav) * (eta_d_est_vec(:,iiuav) - eta0(:) - delta_eta_vec(:,iiuav));
for jjuav = 1:5
    ksi_est_err_tilt_2 = ksi_est_err_tilt_2 + ...
                                        wij(iiuav, jjuav) * ((ksi_d_est_vec(:,iiuav) - delta_ksi_vec(:,iiuav)) - (ksi_d_est_vec(:,jjuav) - delta_ksi_vec(:,jjuav)));
    eta_est_err_tilt_2 = eta_est_err_tilt_2 + ...
                                        wij(iiuav, jjuav) * ((eta_d_est_vec(:,iiuav) - delta_eta_vec(:,iiuav)) - (eta_d_est_vec(:,jjuav) - delta_eta_vec(:,jjuav)));
end

== matlab function sim_tvt_2025_pos_ctrl/cal lumped observation error agent 3 ==
  data: wij input; w0 input; ksi_d_est_vec input; ksi0 input; delta_ksi_vec input; eta_d_est_vec input; ksi_est_err_tilt_3 output; eta0 input; delta_eta_vec input; eta_est_err_tilt_3 output
function [ksi_est_err_tilt_3, eta_est_err_tilt_3]  = fcn(wij, w0, ksi_d_est_vec, ksi0, delta_ksi_vec, eta_d_est_vec, eta0, delta_eta_vec)
%%%% 计算跟随者期望速度分布式观测器误差
iiuav = 3;
ksi_est_err_tilt_3 = w0(iiuav, iiuav) * (ksi_d_est_vec(:,iiuav) - ksi0(:) - delta_ksi_vec(:,iiuav));
eta_est_err_tilt_3 = w0(iiuav, iiuav) * (eta_d_est_vec(:,iiuav) - eta0(:) - delta_eta_vec(:,iiuav));
for jjuav = 1:5
    ksi_est_err_tilt_3 = ksi_est_err_tilt_3 + ...
                                        wij(iiuav, jjuav) * ((ksi_d_est_vec(:,iiuav) - delta_ksi_vec(:,iiuav)) - (ksi_d_est_vec(:,jjuav) - delta_ksi_vec(:,jjuav)));
    eta_est_err_tilt_3 = eta_est_err_tilt_3 + ...
                                        wij(iiuav, jjuav) * ((eta_d_est_vec(:,iiuav) - delta_eta_vec(:,iiuav)) - (eta_d_est_vec(:,jjuav) - delta_eta_vec(:,jjuav)));
end

== matlab function sim_tvt_2025_pos_ctrl/cal lumped observation error agent 4 ==
  data: wij input; w0 input; ksi_d_est_vec input; ksi0 input; delta_ksi_vec input; eta_d_est_vec input; ksi_est_err_tilt_4 output; eta0 input; delta_eta_vec input; eta_est_err_tilt_4 output
function [ksi_est_err_tilt_4, eta_est_err_tilt_4]  = fcn(wij, w0, ksi_d_est_vec, ksi0, delta_ksi_vec, eta_d_est_vec, eta0, delta_eta_vec)
%%%% 计算跟随者期望速度分布式观测器误差
iiuav = 4;
ksi_est_err_tilt_4 = w0(iiuav, iiuav) * (ksi_d_est_vec(:,iiuav) - ksi0(:) - delta_ksi_vec(:,iiuav));
eta_est_err_tilt_4 = w0(iiuav, iiuav) * (eta_d_est_vec(:,iiuav) - eta0(:) - delta_eta_vec(:,iiuav));
for jjuav = 1:5
    ksi_est_err_tilt_4 = ksi_est_err_tilt_4 + ...
                                        wij(iiuav, jjuav) * ((ksi_d_est_vec(:,iiuav) - delta_ksi_vec(:,iiuav)) - (ksi_d_est_vec(:,jjuav) - delta_ksi_vec(:,jjuav)));
    eta_est_err_tilt_4 = eta_est_err_tilt_4 + ...
                                        wij(iiuav, jjuav) * ((eta_d_est_vec(:,iiuav) - delta_eta_vec(:,iiuav)) - (eta_d_est_vec(:,jjuav) - delta_eta_vec(:,jjuav)));
end

== matlab function sim_tvt_2025_pos_ctrl/cal lumped observation error agent 5 ==
  data: wij input; w0 input; ksi_d_est_vec input; ksi0 input; delta_ksi_vec input; eta_d_est_vec input; ksi_est_err_tilt_5 output; eta0 input; delta_eta_vec input; eta_est_err_tilt_5 output
function [ksi_est_err_tilt_5, eta_est_err_tilt_5]  = fcn(wij, w0, ksi_d_est_vec, ksi0, delta_ksi_vec, eta_d_est_vec, eta0, delta_eta_vec)
%%%% 计算跟随者期望速度分布式观测器误差
iiuav = 5;
ksi_est_err_tilt_5 = w0(iiuav, iiuav) * (ksi_d_est_vec(:,iiuav) - ksi0(:) - delta_ksi_vec(:,iiuav));
eta_est_err_tilt_5 = w0(iiuav, iiuav) * (eta_d_est_vec(:,iiuav) - eta0(:) - delta_eta_vec(:,iiuav));
for jjuav = 1:5
    ksi_est_err_tilt_5 = ksi_est_err_tilt_5 + ...
                                        wij(iiuav, jjuav) * ((ksi_d_est_vec(:,iiuav) - delta_ksi_vec(:,iiuav)) - (ksi_d_est_vec(:,jjuav) - delta_ksi_vec(:,jjuav)));
    eta_est_err_tilt_5 = eta_est_err_tilt_5 + ...
                                        wij(iiuav, jjuav) * ((eta_d_est_vec(:,iiuav) - delta_eta_vec(:,iiuav)) - (eta_d_est_vec(:,jjuav) - delta_eta_vec(:,jjuav)));
end

== matlab function sim_tvt_2025_pos_ctrl/cal follower desire position estimate error ==
  data: ksi_d_est_vec input; ksi_est_err output; ksi0 input; delta_ksi_vec input
function ksi_est_err  = fcn(ksi_d_est_vec, ksi0, delta_ksi_vec)
%%%% 计算跟随者期望位置分布式观测器误差
ksi_est_err = ksi_d_est_vec - repmat(ksi0, 1, 5) - delta_ksi_vec;

== matlab function sim_tvt_2025_pos_ctrl/update sigmai agent 4 ==
  data: kai0 input; lam0 input; eps0 input; d_sigmai_4 output; Wij input; Mii input; tsim input; u0 input; beta_hat_vec input; rho_hat_vec input; Phi_sec_sigma_vec input
function d_sigmai_4 = fcn(kai0, lam0, eps0, Wij, Mii, tsim, u0, beta_hat_vec, rho_hat_vec, Phi_sec_sigma_vec)
%%%% 求解分布式观测器变量
iiuav = 4;
err_rho = Mii(iiuav, iiuav) * ( rho_hat_vec(:,iiuav) - u0(:) );
for jjuav = 1:5
    err_rho = err_rho + Wij(iiuav, jjuav) * ( rho_hat_vec(:,iiuav) - rho_hat_vec(:,jjuav) );
end
d_sigmai_4 = -inv( Phi_sec_sigma_vec(:,:,iiuav) ) * ( ( kai0(:) ./ lam0(:) ) .* err_rho(:) ...
                                + ( beta_hat_vec(iiuav) ./ lam0(:) ) .* tanh( err_rho(:) ./ exp( -eps0 * tsim ) ) );

== matlab function sim_tvt_2025_pos_ctrl/cal theta_eta_est_err_tilt agent 1 ==
  data: alfa_theta input; eta_est_err_squ_1_node_1 input; theta_eta_est_err_tilt_1_1 output; eta_est_err_squ_2_node_1 input; eta_est_err_tilt_vec input; theta_eta_est_err_tilt_2_1 output
function [theta_eta_est_err_tilt_1_1, theta_eta_est_err_tilt_2_1] = fcn(alfa_theta, eta_est_err_squ_1_node_1, eta_est_err_squ_2_node_1, eta_est_err_tilt_vec)
%%%% 计算平滑递增函数
iiuav = 1;
theta_eta_est_err_tilt_1_1 = eta_est_err_squ_1_node_1(:) .* ( -1 + 2 ./ ( 1 + exp( -alfa_theta .* eta_est_err_tilt_vec(:,iiuav) ) ) );
theta_eta_est_err_tilt_2_1 = eta_est_err_squ_2_node_1(:) .* ( -1 + 2 ./ ( 1 + exp( -alfa_theta .* eta_est_err_tilt_vec(:,iiuav) ) ) );

== matlab function sim_tvt_2025_pos_ctrl/cal theta_eta_est_err_tilt agent 2 ==
  data: alfa_theta input; eta_est_err_squ_1_node_2 input; theta_eta_est_err_tilt_1_2 output; eta_est_err_squ_2_node_2 input; eta_est_err_tilt_vec input; theta_eta_est_err_tilt_2_2 output
function [theta_eta_est_err_tilt_1_2, theta_eta_est_err_tilt_2_2] = fcn(alfa_theta, eta_est_err_squ_1_node_2, eta_est_err_squ_2_node_2, eta_est_err_tilt_vec)
%%%% 计算平滑递增函数
iiuav = 2;
theta_eta_est_err_tilt_1_2 = eta_est_err_squ_1_node_2(:) .* ( -1 + 2 ./ ( 1 + exp( -alfa_theta .* eta_est_err_tilt_vec(:,iiuav) ) ) );
theta_eta_est_err_tilt_2_2 = eta_est_err_squ_2_node_2(:) .* ( -1 + 2 ./ ( 1 + exp( -alfa_theta .* eta_est_err_tilt_vec(:,iiuav) ) ) );

== matlab function sim_tvt_2025_pos_ctrl/cal theta_eta_est_err_tilt agent 3 ==
  data: alfa_theta input; eta_est_err_squ_1_node_3 input; theta_eta_est_err_tilt_1_3 output; eta_est_err_squ_2_node_3 input; eta_est_err_tilt_vec input; theta_eta_est_err_tilt_2_3 output
function [theta_eta_est_err_tilt_1_3, theta_eta_est_err_tilt_2_3] = fcn(alfa_theta, eta_est_err_squ_1_node_3, eta_est_err_squ_2_node_3, eta_est_err_tilt_vec)
%%%% 计算平滑递增函数
iiuav = 3;
theta_eta_est_err_tilt_1_3 = eta_est_err_squ_1_node_3(:) .* ( -1 + 2 ./ ( 1 + exp( -alfa_theta .* eta_est_err_tilt_vec(:,iiuav) ) ) );
theta_eta_est_err_tilt_2_3 = eta_est_err_squ_2_node_3(:) .* ( -1 + 2 ./ ( 1 + exp( -alfa_theta .* eta_est_err_tilt_vec(:,iiuav) ) ) );

== matlab function sim_tvt_2025_pos_ctrl/cal theta_eta_est_err_tilt agent 4 ==
  data: alfa_theta input; eta_est_err_squ_1_node_4 input; theta_eta_est_err_tilt_1_4 output; eta_est_err_squ_2_node_4 input; eta_est_err_tilt_vec input; theta_eta_est_err_tilt_2_4 output
function [theta_eta_est_err_tilt_1_4, theta_eta_est_err_tilt_2_4] = fcn(alfa_theta, eta_est_err_squ_1_node_4, eta_est_err_squ_2_node_4, eta_est_err_tilt_vec)
%%%% 计算平滑递增函数
iiuav = 4;
theta_eta_est_err_tilt_1_4 = eta_est_err_squ_1_node_4(:) .* ( -1 + 2 ./ ( 1 + exp( -alfa_theta .* eta_est_err_tilt_vec(:,iiuav) ) ) );
theta_eta_est_err_tilt_2_4 = eta_est_err_squ_2_node_4(:) .* ( -1 + 2 ./ ( 1 + exp( -alfa_theta .* eta_est_err_tilt_vec(:,iiuav) ) ) );

== matlab function sim_tvt_2025_pos_ctrl/cal theta_eta_est_err_tilt agent 5 ==
  data: alfa_theta input; eta_est_err_squ_1_node_5 input; theta_eta_est_err_tilt_1_5 output; eta_est_err_squ_2_node_5 input; eta_est_err_tilt_vec input; theta_eta_est_err_tilt_2_5 output
function [theta_eta_est_err_tilt_1_5, theta_eta_est_err_tilt_2_5] = fcn(alfa_theta, eta_est_err_squ_1_node_5, eta_est_err_squ_2_node_5, eta_est_err_tilt_vec)
%%%% 计算平滑递增函数
iiuav = 5;
theta_eta_est_err_tilt_1_5 = eta_est_err_squ_1_node_5(:) .* ( -1 + 2 ./ ( 1 + exp( -alfa_theta .* eta_est_err_tilt_vec(:,iiuav) ) ) );
theta_eta_est_err_tilt_2_5 = eta_est_err_squ_2_node_5(:) .* ( -1 + 2 ./ ( 1 + exp( -alfa_theta .* eta_est_err_tilt_vec(:,iiuav) ) ) );

== matlab function sim_tvt_2025_pos_ctrl/cal theta_ksi_est_err_tilt agent 1 ==
  data: alfa_theta input; ksi_est_err_squ_1_node_1 input; theta_ksi_est_err_tilt_1_1 output; ksi_est_err_squ_2_node_1 input; ksi_est_err_tilt_vec input; theta_ksi_est_err_tilt_2_1 output
function [theta_ksi_est_err_tilt_1_1, theta_ksi_est_err_tilt_2_1] = fcn(alfa_theta, ksi_est_err_squ_1_node_1, ksi_est_err_squ_2_node_1, ksi_est_err_tilt_vec)
%%%% 计算平滑递增函数
iiuav = 1;
theta_ksi_est_err_tilt_1_1 = ksi_est_err_squ_1_node_1(:) .* ( -1 + 2 ./ ( 1 + exp( -alfa_theta .* ksi_est_err_tilt_vec(:,iiuav) ) ) );
theta_ksi_est_err_tilt_2_1 = ksi_est_err_squ_2_node_1(:) .* ( -1 + 2 ./ ( 1 + exp( -alfa_theta .* ksi_est_err_tilt_vec(:,iiuav) ) ) );

== matlab function sim_tvt_2025_pos_ctrl/cal theta_ksi_est_err_tilt agent 2 ==
  data: alfa_theta input; ksi_est_err_squ_1_node_2 input; theta_ksi_est_err_tilt_1_2 output; ksi_est_err_squ_2_node_2 input; ksi_est_err_tilt_vec input; theta_ksi_est_err_tilt_2_2 output
function [theta_ksi_est_err_tilt_1_2, theta_ksi_est_err_tilt_2_2] = fcn(alfa_theta, ksi_est_err_squ_1_node_2, ksi_est_err_squ_2_node_2, ksi_est_err_tilt_vec)
%%%% 计算平滑递增函数
iiuav = 2;
theta_ksi_est_err_tilt_1_2 = ksi_est_err_squ_1_node_2(:) .* ( -1 + 2 ./ ( 1 + exp( -alfa_theta .* ksi_est_err_tilt_vec(:,iiuav) ) ) );
theta_ksi_est_err_tilt_2_2 = ksi_est_err_squ_2_node_2(:) .* ( -1 + 2 ./ ( 1 + exp( -alfa_theta .* ksi_est_err_tilt_vec(:,iiuav) ) ) );

== matlab function sim_tvt_2025_pos_ctrl/cal theta_ksi_est_err_tilt agent 3 ==
  data: alfa_theta input; ksi_est_err_squ_1_node_3 input; theta_ksi_est_err_tilt_1_3 output; ksi_est_err_squ_2_node_3 input; ksi_est_err_tilt_vec input; theta_ksi_est_err_tilt_2_3 output
function [theta_ksi_est_err_tilt_1_3, theta_ksi_est_err_tilt_2_3] = fcn(alfa_theta, ksi_est_err_squ_1_node_3, ksi_est_err_squ_2_node_3, ksi_est_err_tilt_vec)
%%%% 计算平滑递增函数
iiuav = 3;
theta_ksi_est_err_tilt_1_3 = ksi_est_err_squ_1_node_3(:) .* ( -1 + 2 ./ ( 1 + exp( -alfa_theta .* ksi_est_err_tilt_vec(:,iiuav) ) ) );
theta_ksi_est_err_tilt_2_3 = ksi_est_err_squ_2_node_3(:) .* ( -1 + 2 ./ ( 1 + exp( -alfa_theta .* ksi_est_err_tilt_vec(:,iiuav) ) ) );

== matlab function sim_tvt_2025_pos_ctrl/cal theta_ksi_est_err_tilt agent 4 ==
  data: alfa_theta input; ksi_est_err_squ_1_node_4 input; theta_ksi_est_err_tilt_1_4 output; ksi_est_err_squ_2_node_4 input; ksi_est_err_tilt_vec input; theta_ksi_est_err_tilt_2_4 output
function [theta_ksi_est_err_tilt_1_4, theta_ksi_est_err_tilt_2_4] = fcn(alfa_theta, ksi_est_err_squ_1_node_4, ksi_est_err_squ_2_node_4, ksi_est_err_tilt_vec)
%%%% 计算平滑递增函数
iiuav = 4;
theta_ksi_est_err_tilt_1_4 = ksi_est_err_squ_1_node_4(:) .* ( -1 + 2 ./ ( 1 + exp( -alfa_theta .* ksi_est_err_tilt_vec(:,iiuav) ) ) );
theta_ksi_est_err_tilt_2_4 = ksi_est_err_squ_2_node_4(:) .* ( -1 + 2 ./ ( 1 + exp( -alfa_theta .* ksi_est_err_tilt_vec(:,iiuav) ) ) );

== matlab function sim_tvt_2025_pos_ctrl/cal theta_ksi_est_err_tilt agent 5 ==
  data: alfa_theta input; ksi_est_err_squ_1_node_5 input; theta_ksi_est_err_tilt_1_5 output; ksi_est_err_squ_2_node_5 input; ksi_est_err_tilt_vec input; theta_ksi_est_err_tilt_2_5 output
function [theta_ksi_est_err_tilt_1_5, theta_ksi_est_err_tilt_2_5] = fcn(alfa_theta, ksi_est_err_squ_1_node_5, ksi_est_err_squ_2_node_5, ksi_est_err_tilt_vec)
%%%% 计算平滑递增函数
iiuav = 5;
theta_ksi_est_err_tilt_1_5 = ksi_est_err_squ_1_node_5(:) .* ( -1 + 2 ./ ( 1 + exp( -alfa_theta .* ksi_est_err_tilt_vec(:,iiuav) ) ) );
theta_ksi_est_err_tilt_2_5 = ksi_est_err_squ_2_node_5(:) .* ( -1 + 2 ./ ( 1 + exp( -alfa_theta .* ksi_est_err_tilt_vec(:,iiuav) ) ) );

== matlab function sim_tvt_2025_pos_ctrl/cal follower desire velocity estimate error ==
  data: eta_d_est_vec input; eta_est_err output; eta0 input; delta_eta_vec input
function eta_est_err  = fcn(eta_d_est_vec, eta0, delta_eta_vec)
%%%% 计算跟随者期望速度分布式观测器误差
eta_est_err = eta_d_est_vec - repmat(eta0, 1, 5) - delta_eta_vec;

== matlab function sim_tvt_2025_pos_ctrl/choose eta_est_err_tilt 1 ==
  data: x input; y output
function y = fcn(x)
iiuav = 1;
y = x(:,iiuav);

== matlab function sim_tvt_2025_pos_ctrl/choose eta_est_err_tilt 10 ==
  data: x input; y output
function y = fcn(x)
iiuav = 5;
y = x(:,iiuav);

== matlab function sim_tvt_2025_pos_ctrl/choose eta_est_err_tilt 11 ==
  data: x input; y output
function y = fcn(x)
iiuav = 1;
y = x(:,iiuav);

== matlab function sim_tvt_2025_pos_ctrl/cal vel_bar_i agent 1 ==
  data: eta_i_vec input; d_phi_vec input; vel_bar_1 output
function vel_bar_1 = fcn(eta_i_vec, d_phi_vec)
%%%% 计算辅助速度向量
iiuav = 1;
vel_bar_1 = eta_i_vec(:,iiuav) - d_phi_vec(:,iiuav);

== matlab function sim_tvt_2025_pos_ctrl/cal vel_bar_i agent 2 ==
  data: eta_i_vec input; d_phi_vec input; vel_bar_2 output
function vel_bar_2 = fcn(eta_i_vec, d_phi_vec)
%%%% 计算辅助速度向量
iiuav = 2;
vel_bar_2 = eta_i_vec(:,iiuav) - d_phi_vec(:,iiuav);

== matlab function sim_tvt_2025_pos_ctrl/cal vel_bar_i agent 3 ==
  data: eta_i_vec input; d_phi_vec input; vel_bar_3 output
function vel_bar_3 = fcn(eta_i_vec, d_phi_vec)
%%%% 计算辅助速度向量
iiuav = 3;
vel_bar_3 = eta_i_vec(:,iiuav) - d_phi_vec(:,iiuav);

== matlab function sim_tvt_2025_pos_ctrl/update sigmai agent 5 ==
  data: kai0 input; lam0 input; eps0 input; d_sigmai_5 output; Wij input; Mii input; tsim input; u0 input; beta_hat_vec input; rho_hat_vec input; Phi_sec_sigma_vec input
function d_sigmai_5 = fcn(kai0, lam0, eps0, Wij, Mii, tsim, u0, beta_hat_vec, rho_hat_vec, Phi_sec_sigma_vec)
%%%% 求解分布式观测器变量
iiuav = 5;
err_rho = Mii(iiuav, iiuav) * ( rho_hat_vec(:,iiuav) - u0(:) );
for jjuav = 1:5
    err_rho = err_rho + Wij(iiuav, jjuav) * ( rho_hat_vec(:,iiuav) - rho_hat_vec(:,jjuav) );
end
d_sigmai_5 = -inv( Phi_sec_sigma_vec(:,:,iiuav) ) * ( ( kai0(:) ./ lam0(:) ) .* err_rho(:) ...
                                + ( beta_hat_vec(iiuav) ./ lam0(:) ) .* tanh( err_rho(:) ./ exp( -eps0 * tsim ) ) );

== matlab function sim_tvt_2025_pos_ctrl/cal vel_bar_i agent 4 ==
  data: eta_i_vec input; d_phi_vec input; vel_bar_4 output
function vel_bar_4 = fcn(eta_i_vec, d_phi_vec)
%%%% 计算辅助速度向量
iiuav = 4;
vel_bar_4 = eta_i_vec(:,iiuav) - d_phi_vec(:,iiuav);

== matlab function sim_tvt_2025_pos_ctrl/cal vel_bar_i agent 5 ==
  data: eta_i_vec input; d_phi_vec input; vel_bar_5 output
function vel_bar_5 = fcn(eta_i_vec, d_phi_vec)
%%%% 计算辅助速度向量
iiuav = 5;
vel_bar_5 = eta_i_vec(:,iiuav) - d_phi_vec(:,iiuav);

== matlab function sim_tvt_2025_pos_ctrl/combine vel_bar_i ==
  data: vel_bar_1 input; vel_bar_vec output; vel_bar_2 input; vel_bar_3 input; vel_bar_4 input; vel_bar_5 input
function vel_bar_vec  = fcn(vel_bar_1, vel_bar_2, vel_bar_3, vel_bar_4, vel_bar_5)
%%%% 合并辅助速度向量
vel_bar_vec = zeros(3,5);
vel_bar_vec(:,1) = vel_bar_1(:);
vel_bar_vec(:,2) = vel_bar_2(:);
vel_bar_vec(:,3) = vel_bar_3(:);
vel_bar_vec(:,4) = vel_bar_4(:);
vel_bar_vec(:,5) = vel_bar_5(:);

== matlab function sim_tvt_2025_pos_ctrl/choose eta_est_err_tilt 18 ==
  data: x input; y output
function y = fcn(x)
iiuav = 4;
y = x(:,iiuav);

== matlab function sim_tvt_2025_pos_ctrl/choose eta_est_err_tilt 19 ==
  data: x input; y output
function y = fcn(x)
iiuav = 4;
y = x(:,iiuav);

== matlab function sim_tvt_2025_pos_ctrl/choose eta_est_err_tilt 2 ==
  data: x input; y output
function y = fcn(x)
iiuav = 1;
y = x(:,iiuav);

== matlab function sim_tvt_2025_pos_ctrl/choose eta_est_err_tilt 20 ==
  data: x input; y output
function y = fcn(x)
iiuav = 5;
y = x(:,iiuav);

== matlab function sim_tvt_2025_pos_ctrl/choose eta_est_err_tilt 3 ==
  data: x input; y output
function y = fcn(x)
iiuav = 2;
y = x(:,iiuav);

== matlab function sim_tvt_2025_pos_ctrl/choose eta_est_err_tilt 4 ==
  data: x input; y output
function y = fcn(x)
iiuav = 2;
y = x(:,iiuav);

== matlab function sim_tvt_2025_pos_ctrl/choose eta_est_err_tilt 5 ==
  data: x input; y output
function y = fcn(x)
iiuav = 3;
y = x(:,iiuav);

== matlab function sim_tvt_2025_pos_ctrl/choose eta_est_err_tilt 6 ==
  data: x input; y output
function y = fcn(x)
iiuav = 3;
y = x(:,iiuav);

== matlab function sim_tvt_2025_pos_ctrl/choose eta_est_err_tilt 7 ==
  data: x input; y output
function y = fcn(x)
iiuav = 4;
y = x(:,iiuav);

== matlab function sim_tvt_2025_pos_ctrl/choose eta_est_err_tilt 8 ==
  data: x input; y output
function y = fcn(x)
iiuav = 4;
y = x(:,iiuav);

== matlab function sim_tvt_2025_pos_ctrl/choose eta_est_err_tilt 9 ==
  data: x input; y output
function y = fcn(x)
iiuav = 5;
y = x(:,iiuav);

== matlab function sim_tvt_2025_pos_ctrl/combine follower desire velocity estimaters ==
  data: eta_d_est_1 input; eta_d_est_vec output; eta_d_est_2 input; eta_d_est_3 input; eta_d_est_4 input; eta_d_est_5 input
function eta_d_est_vec = fcn(eta_d_est_1, eta_d_est_2, eta_d_est_3, eta_d_est_4, eta_d_est_5)
%%%% 合并领导者位置观测器输出结果
eta_d_est_vec = [eta_d_est_1(:), eta_d_est_2(:), eta_d_est_3(:), eta_d_est_4(:), eta_d_est_5(:)];

== matlab function sim_tvt_2025_pos_ctrl/combine Phi_sec_sigma_i ==
  data: Phi_sec_sigma_1 input; Phi_sec_sigma_vec output; Phi_sec_sigma_2 input; Phi_sec_sigma_3 input; Phi_sec_sigma_4 input; Phi_sec_sigma_5 input
function Phi_sec_sigma_vec  = fcn(Phi_sec_sigma_1, Phi_sec_sigma_2, Phi_sec_sigma_3, Phi_sec_sigma_4, Phi_sec_sigma_5)
%%%% 合并领导者位置观测器输出结果
Phi_sec_sigma_vec = zeros(3,3,5);
Phi_sec_sigma_vec(:,:,1) = Phi_sec_sigma_1;
Phi_sec_sigma_vec(:,:,2) = Phi_sec_sigma_2;
Phi_sec_sigma_vec(:,:,3) = Phi_sec_sigma_3;
Phi_sec_sigma_vec(:,:,4) = Phi_sec_sigma_4;
Phi_sec_sigma_vec(:,:,5) = Phi_sec_sigma_5;

== matlab function sim_tvt_2025_pos_ctrl/combine lumped follower observation error  ==
  data: ksi_est_err_tilt_1 input; ksi_est_err_tilt_2 input; ksi_est_err_tilt_3 input; ksi_est_err_tilt_4 input; ksi_est_err_tilt_5 input; ksi_est_err_tilt_vec output; eta_est_err_tilt_1 input; eta_est_err_tilt_vec output; eta_est_err_tilt_2 input; eta_est_err_tilt_3 input; eta_est_err_tilt_4 input; eta_est_err_tilt_5 input
function [ksi_est_err_tilt_vec, eta_est_err_tilt_vec]  = fcn(ksi_est_err_tilt_1, ksi_est_err_tilt_2, ksi_est_err_tilt_3, ksi_est_err_tilt_4, ksi_est_err_tilt_5, ...
                                                                                                        eta_est_err_tilt_1, eta_est_err_tilt_2, eta_est_err_tilt_3, eta_est_err_tilt_4, eta_est_err_tilt_5)
%%%% 合并领导者位置观测器输出结果
ksi_est_err_tilt_vec = [ksi_est_err_tilt_1, ksi_est_err_tilt_2, ksi_est_err_tilt_3, ksi_est_err_tilt_4, ksi_est_err_tilt_5];
eta_est_err_tilt_vec = [eta_est_err_tilt_1, eta_est_err_tilt_2, eta_est_err_tilt_3, eta_est_err_tilt_4, eta_est_err_tilt_5];
